simulink model "HPF"  (R2023a)
settings: Solver=VariableStepAuto  StartTime=0.0  StopTime=10.0  RelTol=1e-3
settings Model: Creator=洲  LastModifiedBy=洲

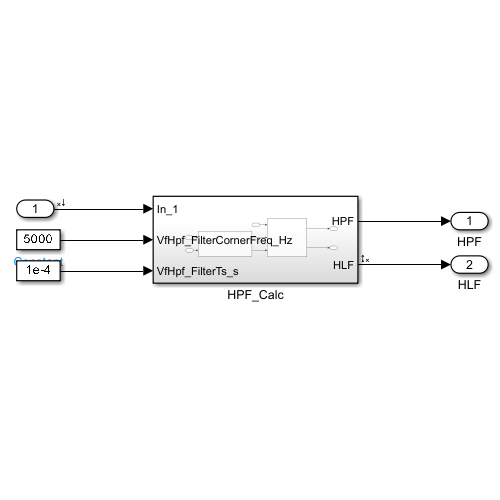
[thumbnail: Simulink's stored preview of the top-level diagram]
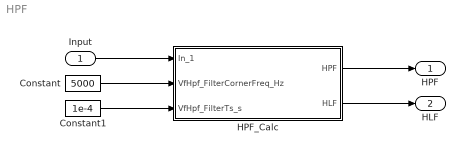
== system HPF ==
  Input : Inport
  Constant : Constant  Value=5000
  Constant1 : Constant  Value=1e-4
  HPF_Calc : Subsystem
  HPF : Outport
  HLF : Outport  Port=2
  wires:
  Input/1 -> HPF_Calc/1(In_1)
  Constant/1 -> HPF_Calc/2(VfHpf_FilterCornerFreq_Hz)
  Constant1/1 -> HPF_Calc/3(VfHpf_FilterTs_s)
  HPF_Calc/1(HPF) -> HPF/1
  HPF_Calc/2(HLF) -> HLF/1

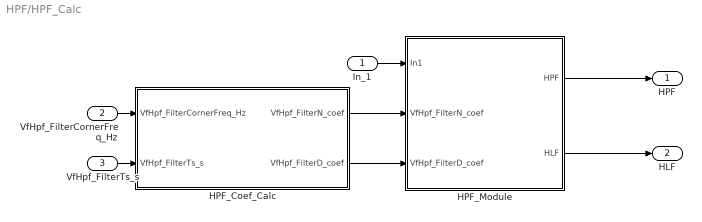
== system HPF/HPF_Calc ==
  In_1 : Inport
  VfHpf_FilterCornerFreq_Hz : Inport  Port=2
  VfHpf_FilterTs_s : Inport  Port=3
  HPF_Coef_Calc : Subsystem
  HPF_Module : Subsystem
  HPF : Outport
  HLF : Outport  Port=2
  wires:
  In_1/1 -> HPF_Module/1(In1)
  HPF_Coef_Calc/1(VfHpf_FilterN_coef) -> HPF_Module/2(VfHpf_FilterN_coef)
  HPF_Module/1(HPF) -> HPF/1
  HPF_Coef_Calc/2(VfHpf_FilterD_coef) -> HPF_Module/3(VfHpf_FilterD_coef)
  VfHpf_FilterCornerFreq_Hz/1 -> HPF_Coef_Calc/1(VfHpf_FilterCornerFreq_Hz)
  VfHpf_FilterTs_s/1 -> HPF_Coef_Calc/2(VfHpf_FilterTs_s)
  HPF_Module/2(HLF) -> HLF/1

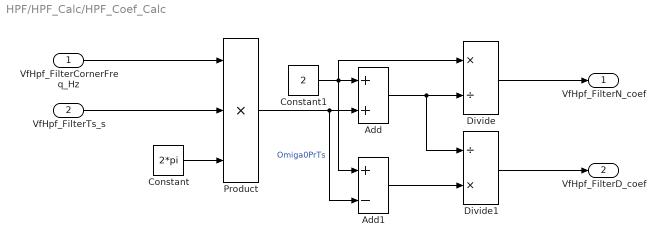
== system HPF/HPF_Calc/HPF_Coef_Calc ==
  VfHpf_FilterCornerFreq_Hz : Inport
  VfHpf_FilterTs_s : Inport  Port=2
  Add : Sum
  Add1 : Sum  Inputs=+-
  Constant : Constant  Value=2*pi  OutDataTypeStr=single
  Constant1 : Constant  Value=2  OutDataTypeStr=single
  Divide : Product  Inputs=*/
  Divide1 : Product  Inputs=/*
  Product : Product  Inputs=3
  VfHpf_FilterN_coef : Outport
  VfHpf_FilterD_coef : Outport  Port=2
  wires:
  VfHpf_FilterCornerFreq_Hz/1 -> Product/1
  VfHpf_FilterTs_s/1 -> Product/2
  Constant/1 -> Product/3
  Product/1 -> Add1/2, Add/2  "Omiga0PrTs"
  Constant1/1 -> Add1/1, Divide/1, Add/1
  Add/1 -> Divide1/1, Divide/2
  Divide/1 -> VfHpf_FilterN_coef/1
  Add1/1 -> Divide1/2
  Divide1/1 -> VfHpf_FilterD_coef/1

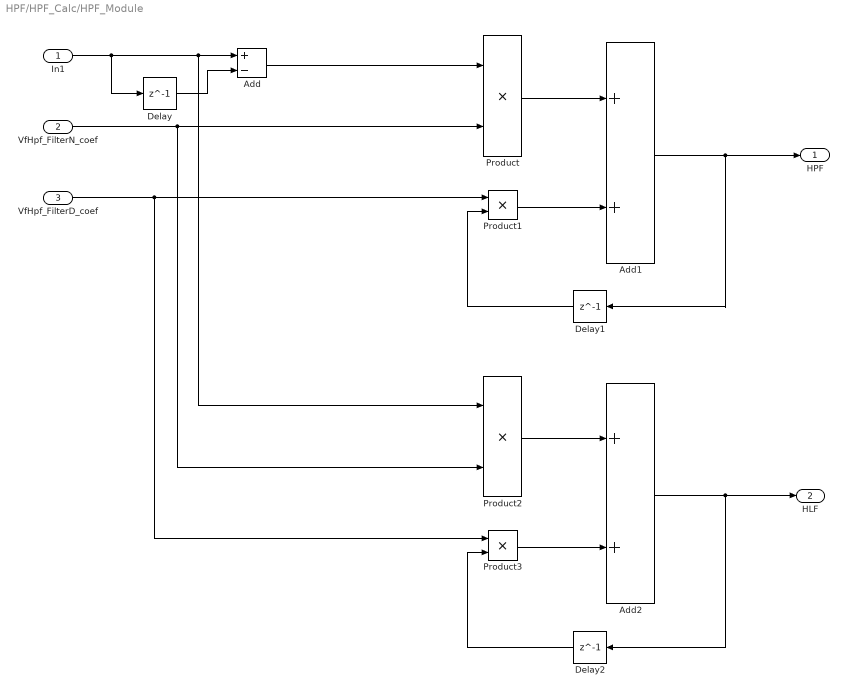
== system HPF/HPF_Calc/HPF_Module ==
  In1 : Inport
  VfHpf_FilterN_coef : Inport  Port=2
  VfHpf_FilterD_coef : Inport  Port=3
  Add : Sum  Inputs=+-
  Add1 : Sum
  Add2 : Sum
  Delay : Delay  DelayLength=1
  Delay1 : Delay  DelayLength=1
  Delay2 : Delay  DelayLength=1
  Product{,1..3} (4 alike) : Product
  HPF : Outport
  HLF : Outport  Port=2
  wires:
  In1/1 -> Delay/1, Product2/1, Add/1
  Delay/1 -> Add/2
  Add/1 -> Product/1
  Product/1 -> Add1/1
  Add1/1 -> Delay1/1, HPF/1
  Product1/1 -> Add1/2
  Delay1/1 -> Product1/2
  VfHpf_FilterD_coef/1 -> Product3/1, Product1/1
  VfHpf_FilterN_coef/1 -> Product2/2, Product/2
  Product2/1 -> Add2/1
  Add2/1 -> HLF/1, Delay2/1
  Delay2/1 -> Product3/2
  Product3/1 -> Add2/2
